simulink model "gm_uz_pmsm_model_3ph_dq"  (R2021b)
settings: Solver=FixedStepAuto  StartTime=0.0  StopTime=0.5  RelTol=1e-3
PreLoadFcn:
  | uz_pmsm_model_init_parameter
undefined symbols (not defined in the file or in its folder): friction_coefficient, inertia, k_i_d, k_p_d, k_p_q, L_d, L_q, polepair, psi_pm, R_1, setpoint_step, simulate_mechanical, simulate_open_loop, static_friction_torque, ts_regler
libraries: hdlmdlgenlib x69, dspsigops x18, slpidlib x2
(part 1 of 2)
settings Model: Creator=ts  LastModifiedBy=valen
settings SolverCC: AlgebraicLoopSolver=TrustRegion  AutoInsertRateTranBlk=on
settings DataIOCC: LimitDataPoints=on  SaveOutput=off  SaveTime=off
settings OptimizationCC: BlockReduction=off  ConditionallyExecuteInputs=off  DefaultParameterBehavior=Inlined  LifeSpan=inf
settings DebuggingCC: AlgebraicLoopMsg=error  InheritedTsInSrcMsg=none  SingleTaskRateTransMsg=error  AllowSymbolicDim=off  StrictBusMsg=ErrorOnBusTreatedAsVector  SFUnexpectedBacktrackingDiag=warning  SFNoUnconditionalDefaultTransitionDiag=warning  SFExecutionAtInitializationDiag=none  SFMachineParentedDataDiag=warning  ArithmeticOperatorsInVariantConditions=warning
settings HardwareCC: ProdBitPerPointer=32  ProdBitPerSizeT=32  ProdBitPerPtrDiffT=32  ProdLargestAtomicFloat=None  ProdIntDivRoundTo=Undefined  ProdEndianess=Unspecified  ProdWordSize=32  ProdHWDeviceType=ASIC/FPGA->ASIC/FPGA  ProdEqTarget=off
settings SFSimCC: SimUseLocalCustomCode=off  CustomCodeUndefinedFunction=UseInterfaceOnly
settings RTWCC: RTWUseLocalCustomCode=off
settings CodeAppCC: StateflowObjectComments=on
settings GRTTargetCC: TargetLangStandard=C89/C90 (ANSI)
settings ConfigComp: CovScope=ReferencedModels  CovMetricSettings=dw  CovSaveCumulativeToWorkspaceVar=on  CovSaveSingleToWorkspaceVar=on  CovExternalEMLEnable=off  CovSFcnEnable=off

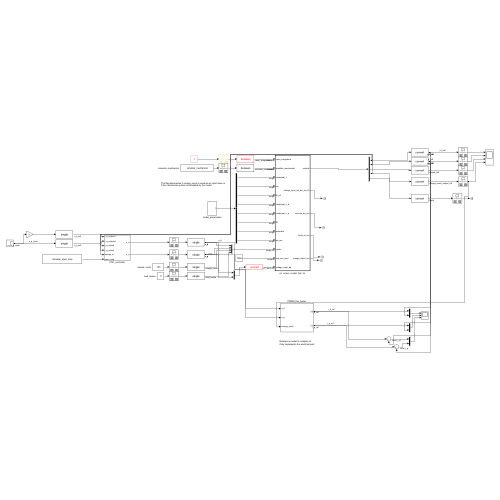
[thumbnail: Simulink's stored preview of the top-level diagram]
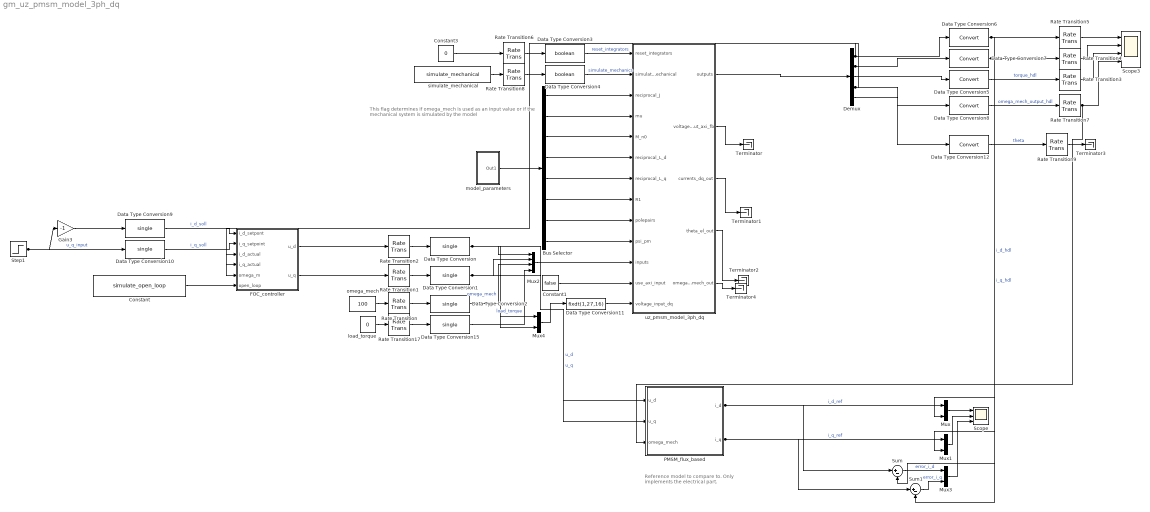
== system gm_uz_pmsm_model_3ph_dq ==
  note: This flag determines if omega_mech is used as an input value or
      | if the mechanical system is simulated by the model
  note: Reference model to compare to.
      | Only implements the electrical part.
  Bus Selector : BusSelector  OutputSignals=1_J,mu,M_R0,1_L_d,1_L_q,R_1,polepair,psi_pm
  Constant : Constant  Value=simulate_open_loop
  Constant1 : Constant  Value=false  OutDataTypeStr=boolean  SampleTime=-1
  Constant3 : Constant  Value=0
  Data Type Conversion{,1..2,9..10,15} (6 alike) : DataTypeConversion  OutDataTypeStr=single
  Data Type Conversion11 : DataTypeConversion  OutDataTypeStr=fixdt(1,27,16)
  Data Type Conversion{5..8,12} (5 alike) : DataTypeConversion
  Data Type Conversion3 : DataTypeConversion  OutDataTypeStr=boolean
  Data Type Conversion4 : DataTypeConversion  OutDataTypeStr=boolean
  Demux : Demux  Outputs=5
  FOC_controller : Subsystem
  Gain3 : Gain  Gain=-1
  Mux{,1,3..4} (4 alike) : Mux  Inputs=2
  Mux2 : Mux
  PMSM_flux_based : Subsystem
  Rate Transition{,1..2,6,8,17} (6 alike) : RateTransition  OutPortSampleTime=ts
  Rate Transition{3..5,7,9} (5 alike) : RateTransition
  Scope : Scope  NumInputPorts=3
  Scope3 : Scope  NumInputPorts=4
  Step1 : Step  Time=0.2  After=setpoint_step  SampleTime=ts_regler
  Sum : Sum  Inputs=|+-
  Sum1 : Sum  Inputs=|+-
  Terminator{,1..4} (5 alike) : Terminator
  load_torque : Constant  Value=0
  model_parameters : Subsystem
  omega_mech : Constant  Value=100
  simulate_mechanical : Constant  Value=simulate_mechanical
  uz_pmsm_model_3ph_dq : Subsystem  TreatAsAtomicUnit=on
  wires:
  uz_pmsm_model_3ph_dq/5(omega_mech_out) -> Terminator4/1
  Rate Transition9/1 -> Terminator3/1
  Data Type Conversion12/1 -> Rate Transition9/1  "theta"
  Demux/5 -> Data Type Conversion12/1
  uz_pmsm_model_3ph_dq/4(theta_el_out) -> Terminator2/1
  uz_pmsm_model_3ph_dq/3(currents_dq_out) -> Terminator1/1
  uz_pmsm_model_3ph_dq/2(voltage_input_dq_out_axi_fb) -> Terminator/1
  Data Type Conversion11/1 -> uz_pmsm_model_3ph_dq/13(voltage_input_dq)
  Mux4/1 -> Data Type Conversion11/1
  Constant1/1 -> uz_pmsm_model_3ph_dq/12(use_axi_input)
  Constant/1 -> FOC_controller/6(open_loop)
  omega_mech/1 -> Rate Transition/1
  FOC_controller/2(u_q) -> Rate Transition1/1
  FOC_controller/1(u_d) -> Rate Transition2/1
  Data Type Conversion10/1 -> FOC_controller/2(i_q_setpoint)  "i_q_soll"
  Data Type Conversion9/1 -> FOC_controller/1(i_d_setpont)  "i_d_soll"
  uz_pmsm_model_3ph_dq/1(outputs) -> Demux/1
  Mux2/1 -> uz_pmsm_model_3ph_dq/11(inputs)
  Data Type Conversion2/1 -> Mux2/3  "omega_mech"
  Data Type Conversion15/1 -> Mux2/4  "load_torque"
  Data Type Conversion1/1 -> Mux2/2, Mux4/2, PMSM_flux_based/2(u_q)  "u_q"
  Data Type Conversion/1 -> PMSM_flux_based/1(u_d), Mux4/1, Mux2/1  "u_d"
  Demux/2 -> Data Type Conversion7/1, FOC_controller/4(i_q_actual)
  Demux/4 -> FOC_controller/5(omega_m), Data Type Conversion8/1
  Demux/1 -> Data Type Conversion6/1, FOC_controller/3(i_d_actual)
  Gain3/1 -> Data Type Conversion9/1
  Demux/3 -> Data Type Conversion5/1
  Step1/1 -> Data Type Conversion10/1, Gain3/1  "u_q_input"
  Mux3/1 -> Scope/3
  Sum1/1 -> Mux3/2  "error_i_q"
  Sum/1 -> Mux3/1  "error_i_d"
  model_parameters/1(Out1) -> Bus Selector/1
  Bus Selector/8 -> uz_pmsm_model_3ph_dq/10(psi_pm)
  Bus Selector/7 -> uz_pmsm_model_3ph_dq/9(polepairs)
  Bus Selector/6 -> uz_pmsm_model_3ph_dq/8(R1)
  Bus Selector/5 -> uz_pmsm_model_3ph_dq/7(reciprocal_L_q)
  Bus Selector/4 -> uz_pmsm_model_3ph_dq/6(reciprocal_L_d)
  Bus Selector/3 -> uz_pmsm_model_3ph_dq/5(M_n0)
  Bus Selector/2 -> uz_pmsm_model_3ph_dq/4(mu)
  Bus Selector/1 -> uz_pmsm_model_3ph_dq/3(reciprocal_J)
  Rate Transition7/1 -> Scope3/4, PMSM_flux_based/3(omega_mech)
  Data Type Conversion8/1 -> Rate Transition7/1  "omega_mech_output_hdl"
  PMSM_flux_based/1(i_d) -> Sum/1, Mux/1  "i_d_ref"
  PMSM_flux_based/2(i_q) -> Sum1/1, Mux1/1  "i_q_ref"
  Mux1/1 -> Scope/2
  Mux/1 -> Scope/1
  Rate Transition17/1 -> Data Type Conversion15/1
  load_torque/1 -> Rate Transition17/1
  Data Type Conversion4/1 -> uz_pmsm_model_3ph_dq/2(simulate_mechanical)  "simulate_mechanics"
  Data Type Conversion3/1 -> uz_pmsm_model_3ph_dq/1(reset_integrators)  "reset_integrators"
  simulate_mechanical/1 -> Rate Transition8/1
  Rate Transition8/1 -> Data Type Conversion4/1
  Constant3/1 -> Rate Transition6/1
  Rate Transition6/1 -> Data Type Conversion3/1
  Rate Transition3/1 -> Scope3/3
  Rate Transition5/1 -> Scope3/1
  Rate Transition4/1 -> Scope3/2
  Data Type Conversion5/1 -> Rate Transition3/1  "torque_hdl"
  Data Type Conversion7/1 -> Mux1/2, Sum1/2, Rate Transition4/1  "i_q_hdl"
  Data Type Conversion6/1 -> Rate Transition5/1, Sum/2, Mux/2  "i_d_hdl"
  Rate Transition2/1 -> Data Type Conversion/1
  Rate Transition1/1 -> Data Type Conversion1/1
  Rate Transition/1 -> Data Type Conversion2/1

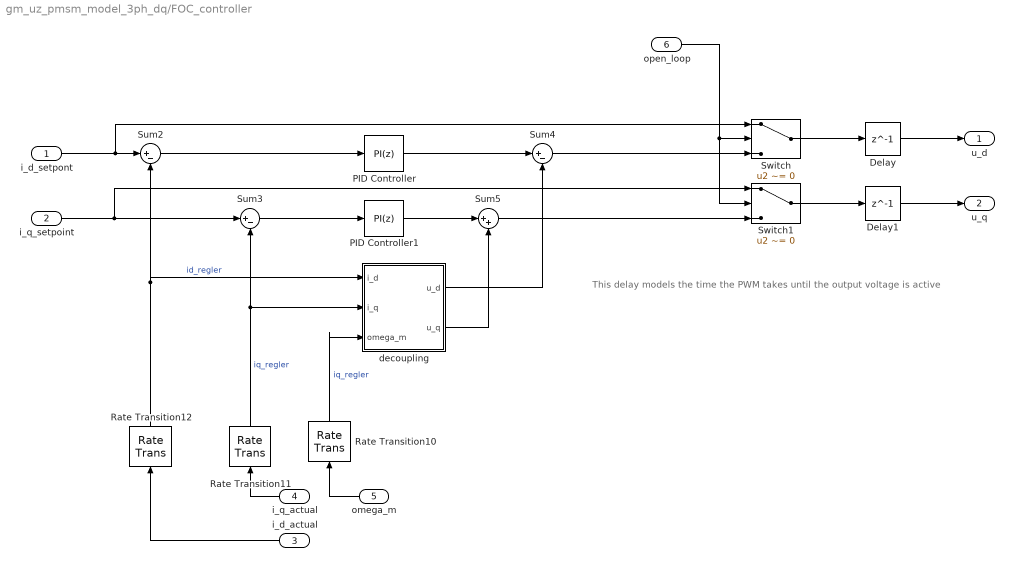
== system gm_uz_pmsm_model_3ph_dq/FOC_controller ==
  note: This delay models the time the PWM takes until the output voltage is active
  i_d_setpont : Inport
  i_q_setpoint : Inport  Port=2
  i_d_actual : Inport  Port=3
  i_q_actual : Inport  Port=4
  omega_m : Inport  Port=5
  open_loop : Inport  Port=6
  Delay : Delay  DelayLength=1
  Delay1 : Delay  DelayLength=1
  PID Controller : slpidlib/PID Controller  Controller=PI  Form=Parallel  TimeDomain=Discrete-time  UseExternalTs=off  SampleTime=-1  IntegratorMethod=Forward Euler  FilterMethod=Forward Euler  ControllerParametersSource=internal  P=k_p_d  I=k_i_d  D=0  UseFilter=on  N=100  TunerSelectOption=Transfer Function Based (PID Tuner App)  InitialConditionSource=internal  InitialConditionForIntegrator=0  InitialConditionForFilter=0  DifferentiatorICPrevScaledInput=0  ExternalReset=none  TrackingMode=off  Kt=1  LimitOutput=off  SatLimitsSource=internal  UpperSaturationLimit=inf  LowerSaturationLimit=-inf  LinearizeAsGain=on  AntiWindupMode=none  Kb=1  POutMin=[]  POutMax=[]  IOutMin=[]  IOutMax=[]  DOutMin=[]  DOutMax=[]  NOutMin=[]  NOutMax=[]  SumOutMin=[]  SumOutMax=[]  SaturationOutMin=[]  SaturationOutMax=[]  PParamMin=[]  PParamMax=[]  IParamMin=[]  IParamMax=[]  DParamMin=[]  DParamMax=[]  NParamMin=[]  NParamMax=[]  KbParamMin=[]  KbParamMax=[]  KtParamMin=[]  KtParamMax=[]  KbOutMin=[]  KbOutMax=[]  KtOutMin=[]  KtOutMax=[]  IntegratorOutMin=[]  IntegratorOutMax=[]  FilterOutMin=[]  FilterOutMax=[]  SumI1OutMin=[]  SumI1OutMax=[]  SumI2OutMin=[]  SumI2OutMax=[]  SumI3OutMin=[]  SumI3OutMax=[]  SumI4OutMin=[]  SumI4OutMax=[]  SumDOutMin=[]  SumDOutMax=[]  DifferentiatorOutMin=[]  DifferentiatorOutMax=[]  FilterDiffOutCoefMin=[]  FilterDiffOutCoefMax=[]  ReciprocalOutMin=[]  ReciprocalOutMax=[]  SumDenOutMin=[]  SumDenOutMax=[]  SumNumOutMin=[]  SumNumOutMax=[]  DivideOutMin=[]  DivideOutMax=[]  UdiffTsProdOutMin=[]  UdiffTsProdOutMax=[]  NTsProdOutMin=[]  NTsProdOutMax=[]  UintegralTsProdOutMin=[]  UintegralTsProdOutMax=[]  UngainTsProdOutMin=[]  UngainTsProdOutMax=[]  IntegratorContinuousStateAttributes=''  IntegratorStateMustResolveToSignalObject=off  IntegratorRTWStateStorageClass=Auto  FilterContinuousStateAttributes=''  FilterStateMustResolveToSignalObject=off  FilterRTWStateStorageClass=Auto  ParallelPVariant=InternalParameters  IdealPVariant=Disabled  IVariant=InternalParameters  DVariant=Disabled  IntegratorVariant=Discrete  SatVariant=Disabled  AWVariant=Passthrough  PCopyVariant=Disabled  TRVariant=Disabled  FdbkBlocksVariant=Forward  IdealPFdbkVariant=Disabled  SatFdbkVariant=Disabled  DerivativeFilterVariant=Disabled  NVariant=Disabled  NCopyVariant=Disabled_SignalSpec  FilterICVariant=Disabled  IntegratorICVariant=InternalICs  ExternalResetVariant=Disabled  TRSumVariant=Passthrough  SumFdbkVariant=Disabled  SumVariant=Sum_PI  TsampFilterVariant=InternalTs  TsampNgainVariant=Passthrough  TsampIntegralVariant=Passthrough  ExternalSaturationOutDataTypeStr=Inherit: Same as second input
  PID Controller1 : slpidlib/PID Controller  Controller=PI  Form=Parallel  TimeDomain=Discrete-time  UseExternalTs=off  SampleTime=-1  IntegratorMethod=Forward Euler  FilterMethod=Forward Euler  ControllerParametersSource=internal  P=k_p_q  I=k_i_d  D=0  UseFilter=on  N=100  TunerSelectOption=Transfer Function Based (PID Tuner App)  InitialConditionSource=internal  InitialConditionForIntegrator=0  InitialConditionForFilter=0  DifferentiatorICPrevScaledInput=0  ExternalReset=none  TrackingMode=off  Kt=1  LimitOutput=off  SatLimitsSource=internal  UpperSaturationLimit=inf  LowerSaturationLimit=-inf  LinearizeAsGain=on  AntiWindupMode=none  Kb=1  POutMin=[]  POutMax=[]  IOutMin=[]  IOutMax=[]  DOutMin=[]  DOutMax=[]  NOutMin=[]  NOutMax=[]  SumOutMin=[]  SumOutMax=[]  SaturationOutMin=[]  SaturationOutMax=[]  PParamMin=[]  PParamMax=[]  IParamMin=[]  IParamMax=[]  DParamMin=[]  DParamMax=[]  NParamMin=[]  NParamMax=[]  KbParamMin=[]  KbParamMax=[]  KtParamMin=[]  KtParamMax=[]  KbOutMin=[]  KbOutMax=[]  KtOutMin=[]  KtOutMax=[]  IntegratorOutMin=[]  IntegratorOutMax=[]  FilterOutMin=[]  FilterOutMax=[]  SumI1OutMin=[]  SumI1OutMax=[]  SumI2OutMin=[]  SumI2OutMax=[]  SumI3OutMin=[]  SumI3OutMax=[]  SumI4OutMin=[]  SumI4OutMax=[]  SumDOutMin=[]  SumDOutMax=[]  DifferentiatorOutMin=[]  DifferentiatorOutMax=[]  FilterDiffOutCoefMin=[]  FilterDiffOutCoefMax=[]  ReciprocalOutMin=[]  ReciprocalOutMax=[]  SumDenOutMin=[]  SumDenOutMax=[]  SumNumOutMin=[]  SumNumOutMax=[]  DivideOutMin=[]  DivideOutMax=[]  UdiffTsProdOutMin=[]  UdiffTsProdOutMax=[]  NTsProdOutMin=[]  NTsProdOutMax=[]  UintegralTsProdOutMin=[]  UintegralTsProdOutMax=[]  UngainTsProdOutMin=[]  UngainTsProdOutMax=[]  IntegratorContinuousStateAttributes=''  IntegratorStateMustResolveToSignalObject=off  IntegratorRTWStateStorageClass=Auto  FilterContinuousStateAttributes=''  FilterStateMustResolveToSignalObject=off  FilterRTWStateStorageClass=Auto  ParallelPVariant=InternalParameters  IdealPVariant=Disabled  IVariant=InternalParameters  DVariant=Disabled  IntegratorVariant=Discrete  SatVariant=Disabled  AWVariant=Passthrough  PCopyVariant=Disabled  TRVariant=Disabled  FdbkBlocksVariant=Forward  IdealPFdbkVariant=Disabled  SatFdbkVariant=Disabled  DerivativeFilterVariant=Disabled  NVariant=Disabled  NCopyVariant=Disabled_SignalSpec  FilterICVariant=Disabled  IntegratorICVariant=InternalICs  ExternalResetVariant=Disabled  TRSumVariant=Passthrough  SumFdbkVariant=Disabled  SumVariant=Sum_PI  TsampFilterVariant=InternalTs  TsampNgainVariant=Passthrough  TsampIntegralVariant=Passthrough  ExternalSaturationOutDataTypeStr=Inherit: Same as second input
  Rate Transition10 : RateTransition  OutPortSampleTime=ts_regler
  Rate Transition11 : RateTransition  OutPortSampleTime=ts_regler
  Rate Transition12 : RateTransition  OutPortSampleTime=ts_regler
  Sum2 : Sum  Inputs=|+-
  Sum3 : Sum  Inputs=|+-
  Sum4 : Sum  Inputs=|+-
  Sum5 : Sum  Inputs=|++
  Switch : Switch  Criteria=u2 ~= 0
  Switch1 : Switch  Criteria=u2 ~= 0
  decoupling : Subsystem
  u_d : Outport
  u_q : Outport  Port=2
  wires:
  Delay1/1 -> u_q/1
  Delay/1 -> u_d/1
  Switch1/1 -> Delay1/1
  Switch/1 -> Delay/1
  decoupling/2(u_q) -> Sum5/2
  decoupling/1(u_d) -> Sum4/2
  Rate Transition10/1 -> decoupling/3(omega_m)  "iq_regler"
  open_loop/1 -> Switch/2, Switch1/2
  i_q_setpoint/1 -> Sum3/1, Switch1/1
  Rate Transition11/1 -> Sum3/2, decoupling/2(i_q)  "iq_regler"
  Rate Transition12/1 -> Sum2/2, decoupling/1(i_d)  "id_regler"
  i_q_actual/1 -> Rate Transition11/1
  Sum3/1 -> PID Controller1/1
  omega_m/1 -> Rate Transition10/1
  Sum5/1 -> Switch1/3
  Sum2/1 -> PID Controller/1
  i_d_setpont/1 -> Sum2/1, Switch/1
  i_d_actual/1 -> Rate Transition12/1
  Sum4/1 -> Switch/3
  PID Controller1/1 -> Sum5/1
  PID Controller/1 -> Sum4/1

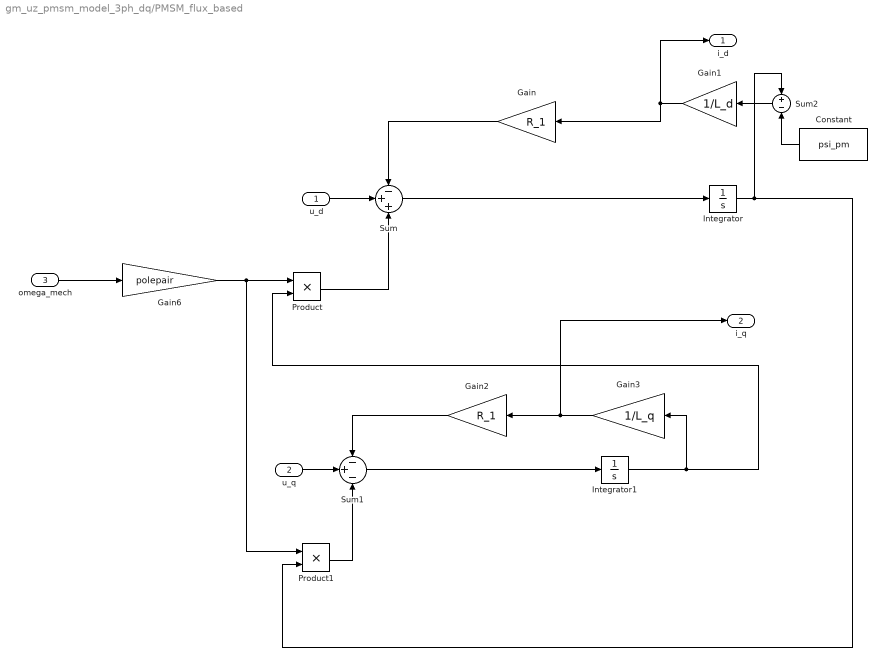
== system gm_uz_pmsm_model_3ph_dq/PMSM_flux_based ==
  u_d : Inport
  u_q : Inport  Port=2
  omega_mech : Inport  Port=3
  Constant : Constant  Value=psi_pm
  Gain : Gain  Gain=R_1
  Gain1 : Gain  Gain=1/L_d
  Gain2 : Gain  Gain=R_1
  Gain3 : Gain  Gain=1/L_q
  Gain6 : Gain  Gain=polepair
  Integrator : Integrator
  Integrator1 : Integrator
  Product : Product
  Product1 : Product
  Sum : Sum  Inputs=-++
  Sum1 : Sum  Inputs=-+-
  Sum2 : Sum  Inputs=+-
  i_d : Outport
  i_q : Outport  Port=2
  wires:
  omega_mech/1 -> Gain6/1
  Gain3/1 -> Gain2/1, i_q/1
  Gain2/1 -> Sum1/1
  Sum1/1 -> Integrator1/1
  Product1/1 -> Sum1/3
  Integrator1/1 -> Product/2, Gain3/1
  Product/1 -> Sum/3
  Gain6/1 -> Product/1, Product1/1
  Gain1/1 -> i_d/1, Gain/1
  Sum2/1 -> Gain1/1
  Constant/1 -> Sum2/2
  Integrator/1 -> Sum2/1, Product1/2
  Gain/1 -> Sum/1
  Sum/1 -> Integrator/1
  u_q/1 -> Sum1/2
  u_d/1 -> Sum/2

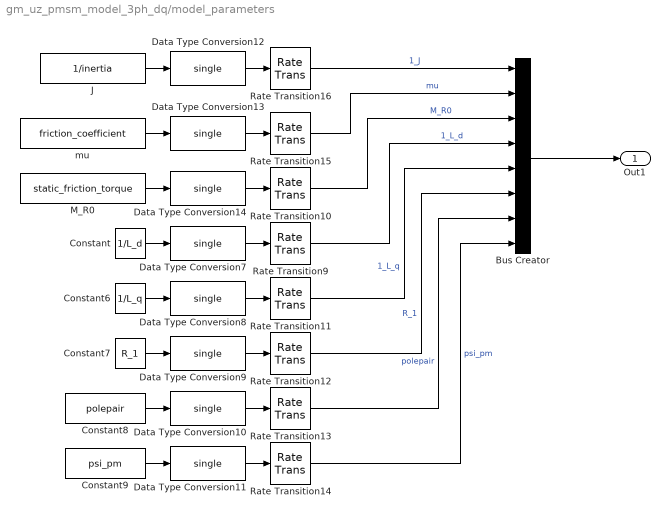
== system gm_uz_pmsm_model_3ph_dq/model_parameters ==
  Bus Creator : BusCreator  Inputs=8
  Constant : Constant  Value=1/L_d
  Constant6 : Constant  Value=1/L_q
  Constant7 : Constant  Value=R_1
  Constant8 : Constant  Value=polepair
  Constant9 : Constant  Value=psi_pm
  Data Type Conversion{7..14} (8 alike) : DataTypeConversion  OutDataTypeStr=single
  J : Constant  Value=1/inertia
  M_R0 : Constant  Value=static_friction_torque
  Rate Transition{9..16} (8 alike) : RateTransition  OutPortSampleTime=ts
  mu : Constant  Value=friction_coefficient
  Out1 : Outport
  wires:
  Constant/1 -> Data Type Conversion7/1
  Constant9/1 -> Data Type Conversion11/1
  Constant7/1 -> Data Type Conversion9/1
  Data Type Conversion13/1 -> Rate Transition15/1
  Rate Transition11/1 -> Bus Creator/5  "1_L_q"
  M_R0/1 -> Data Type Conversion14/1
  mu/1 -> Data Type Conversion13/1
  Data Type Conversion10/1 -> Rate Transition13/1
  Data Type Conversion8/1 -> Rate Transition11/1
  J/1 -> Data Type Conversion12/1
  Rate Transition9/1 -> Bus Creator/4  "1_L_d"
  Constant6/1 -> Data Type Conversion8/1
  Rate Transition15/1 -> Bus Creator/2  "mu"
  Data Type Conversion9/1 -> Rate Transition12/1
  Constant8/1 -> Data Type Conversion10/1
  Data Type Conversion11/1 -> Rate Transition14/1
  Bus Creator/1 -> Out1/1
  Rate Transition13/1 -> Bus Creator/7  "polepair"
  Rate Transition16/1 -> Bus Creator/1  "1_J"
  Rate Transition12/1 -> Bus Creator/6  "R_1"
  Data Type Conversion14/1 -> Rate Transition10/1
  Rate Transition14/1 -> Bus Creator/8  "psi_pm"
  Rate Transition10/1 -> Bus Creator/3  "M_R0"
  Data Type Conversion7/1 -> Rate Transition9/1
  Data Type Conversion12/1 -> Rate Transition16/1

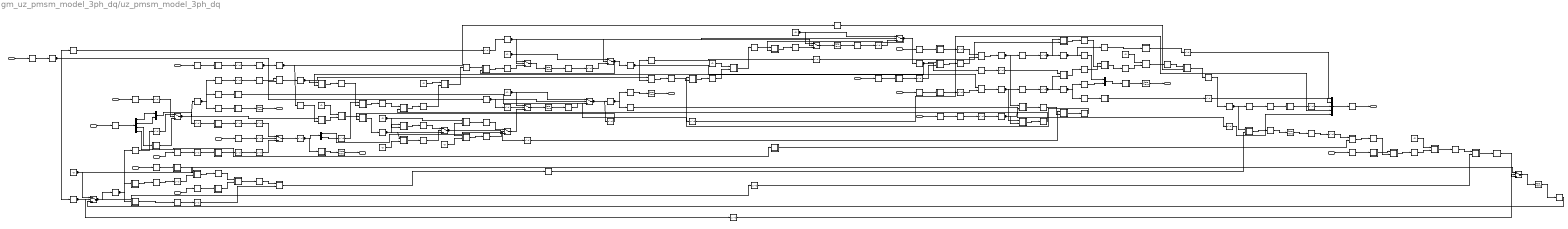
== system gm_uz_pmsm_model_3ph_dq/uz_pmsm_model_3ph_dq ==
  note: https://de.mathworks.com/help/releases/R2021a/hdlcoder/ug/troubleshoot-generate-implementation-model-from-simscape-pmsm.html?searchHighlight=troubleshoot-generate-implementation-model-from-simscape-pmsm&s_tid=doc_srchtitle
  reset_integrators : Inport  OutDataTypeStr=boolean  PortDimensions=1  SampleTime=1e-06
  simulate_mechanical : Inport  Port=2  OutDataTypeStr=boolean  PortDimensions=1  SampleTime=1e-06
  reciprocal_J : Inport  Port=3  OutDataTypeStr=single  PortDimensions=1  SampleTime=1e-06
  mu : Inport  Port=4  OutDataTypeStr=single  PortDimensions=1  SampleTime=1e-06
  M_n0 : Inport  Port=5  OutDataTypeStr=single  PortDimensions=1  SampleTime=1e-06
  reciprocal_L_d : Inport  Port=6  OutDataTypeStr=single  PortDimensions=1  SampleTime=1e-06
  reciprocal_L_q : Inport  Port=7  OutDataTypeStr=single  PortDimensions=1  SampleTime=1e-06
  R1 : Inport  Port=8  OutDataTypeStr=single  PortDimensions=1  SampleTime=1e-06
  polepairs : Inport  Port=9  OutDataTypeStr=single  PortDimensions=1  SampleTime=1e-06
  psi_pm : Inport  Port=10  OutDataTypeStr=single  PortDimensions=1  SampleTime=1e-06
  inputs : Inport  Port=11  OutDataTypeStr=single  PortDimensions=[4]  SampleTime=1e-06
  use_axi_input : Inport  Port=12  OutDataTypeStr=boolean  PortDimensions=1  SampleTime=1e-06
  voltage_input_dq : Inport  Port=13  OutDataTypeStr=fixdt(1, 27, 16)  PortDimensions=[2]  SampleTime=1e-06
  Abs : Subsystem
      mask Display: disp('NFP\nabs');
  Abs_outbuff : hdlmdlgenlib/Buffer
      settings: SourceProductBaseCode=SL
  Compare To Constant1_const : Constant  Value=double(-3.1415927410125732)  OutDataTypeStr=double  SampleTime=1e-08
  Compare To Constant1_relop : Subsystem
      mask Display: disp('NFP\nrelop');
  Compare To Constant1_relop_outbuff : hdlmdlgenlib/Buffer
      settings: SourceProductBaseCode=SL
  Compare To Constant_const : Constant  Value=double(3.1415927410125732)  OutDataTypeStr=double  SampleTime=1e-08
  Compare To Constant_relop : Subsystem
      mask Display: disp('NFP\nrelop');
  Compare To Constant_relop_outbuff : hdlmdlgenlib/Buffer
      settings: SourceProductBaseCode=SL
  Constant : Constant  Value=double(6.283185307179586)  OutDataTypeStr=double  SampleTime=1e-08
  Data Type Conversion1 : Subsystem
      mask Display: disp('NFP\nconv');
  Data Type Conversion10 : Subsystem
      mask Display: disp('NFP\nconv');
  Data Type Conversion10_out1 : hdlmdlgenlib/Buffer
      settings: SourceProductBaseCode=SL
  Data Type Conversion10_out1_in_pipe : Delay  DelayLength=double(7)  InitialCondition=0  SampleTime=1e-08
  Data Type Conversion11 : Subsystem
      mask Display: disp('NFP\nconv');
  Data Type Conversion12 : Subsystem
      mask Display: disp('NFP\nconv');
  Data Type Conversion13 : Subsystem
      mask Display: disp('NFP\nconv');
  Data Type Conversion14 : Subsystem
      mask Display: disp('NFP\nconv');
  Data Type Conversion15 : Subsystem
      mask Display: disp('NFP\nconv');
  Data Type Conversion16 : Subsystem
      mask Display: disp('NFP\nconv');
  Data Type Conversion17 : Subsystem
      mask Display: disp('NFP\nconv');
  Data Type Conversion18 : Subsystem
      mask Display: disp('NFP\nconv');
  Data Type Conversion18_in_pipe : Delay  DelayLength=double(10)  InitialCondition=0  SampleTime=1e-08
  Data Type Conversion18_out_pipe : Delay  DelayLength=double(7)  InitialCondition=0  SampleTime=1e-08
  Data Type Conversion19 : Subsystem
      mask Display: disp('NFP\nconv');
  Data Type Conversion1_in_pipe : Delay  DelayLength=double(10)  InitialCondition=0  SampleTime=1e-08
  Data Type Conversion1_out_pipe : Delay  DelayLength=double(7)  InitialCondition=0  SampleTime=1e-08
  Data Type Conversion2 : Subsystem
      mask Display: disp('NFP\nconv');
  Data Type Conversion20 : Subsystem
      mask Display: disp('NFP\nconv');
  Data Type Conversion21 : Subsystem
      mask Display: disp('NFP\nconv');
  Data Type Conversion3 : Subsystem
      mask Display: disp('NFP\nconv');
  Data Type Conversion4 : Subsystem
      mask Display: disp('NFP\nconv');
  Data Type Conversion5 : Subsystem
      mask Display: disp('NFP\nconv');
  Data Type Conversion6 : Subsystem
      mask Display: disp('NFP\nconv');
  Data Type Conversion6_out1 : hdlmdlgenlib/Buffer
      settings: SourceProductBaseCode=SL
  Data Type Conversion6_out1_in_pipe : Delay  DelayLength=double(7)  InitialCondition=0  SampleTime=1e-08
  Data Type Conversion7 : Subsystem
      mask Display: disp('NFP\nconv');
  Data Type Conversion7_out1_in_pipe : Delay  DelayLength=double(7)  InitialCondition=0  SampleTime=1e-08
  Data Type Conversion8 : Subsystem
      mask Display: disp('NFP\nconv');
  Data Type Conversion8_out1_in_pipe : Delay  DelayLength=double(7)  InitialCondition=0  SampleTime=1e-08
  Data Type Conversion9 : Subsystem
      mask Display: disp('NFP\nconv');
  Data Type Conversion9_out1_in_pipe : Delay  DelayLength=double(7)  InitialCondition=0  SampleTime=1e-08
  Delay : RateTransition  OutPortSampleTimeOpt=Multiple of input port sample time  OutPortSampleTimeMultiple=100
  Delay1_lowered{,1..3} (4 alike) : RateTransition  OutPortSampleTimeOpt=Multiple of input port sample time  OutPortSampleTimeMultiple=100
  Factor : Subsystem
      mask Display: disp('NFP\nmul');
  Factor_const : Constant  Value=double(1.5)  OutDataTypeStr=double  SampleTime=1e-08
  Factor_outbuff : hdlmdlgenlib/Buffer
      settings: SourceProductBaseCode=SL
  From{,1..12} (13 alike) : hdlmdlgenlib/Buffer
      settings: SourceProductBaseCode=SL
  Gain : Subsystem
      mask Display: disp('NFP\nmul');
  Gain1 : Subsystem
      mask Display: disp('NFP\nmul');
  Gain2 : Subsystem
      mask Display: disp('NFP\nmul');
  Gain3 : Subsystem
      mask Display: disp('NFP\nmul');
  Gain_const{,1..3} (4 alike) : Constant  Value=double(1e-06)  OutDataTypeStr=double  SampleTime=1e-08
  Gain_outbuff : hdlmdlgenlib/Buffer
      settings: SourceProductBaseCode=SL
  Gain_outbuff1 : hdlmdlgenlib/Buffer
      settings: SourceProductBaseCode=SL
  Gain_outbuff2 : hdlmdlgenlib/Buffer
      settings: SourceProductBaseCode=SL
  Goto{,1..5} (6 alike) : hdlmdlgenlib/Buffer
      settings: SourceProductBaseCode=SL
  Initial_Val{,1..3} (4 alike) : Constant  Value=double(0)  OutDataTypeStr=double  SampleTime=1e-08
  M_Mi : hdlmdlgenlib/Buffer
      settings: SourceProductBaseCode=SL
  Mux_in_pipe{0..4} (5 alike) : Delay  DelayLength=double(7)  InitialCondition=0  SampleTime=1e-08
  Product : Subsystem
      mask Display: disp('NFP\nmul');
  Product1 : Subsystem
      mask Display: disp('NFP\nmul');
  Product10 : Subsystem
      mask Display: disp('NFP\nmul');
  Product10_outbuff : hdlmdlgenlib/Buffer
      settings: SourceProductBaseCode=SL
  Product11 : Subsystem
      mask Display: disp('NFP\nmul');
  Product11_outbuff : hdlmdlgenlib/Buffer
      settings: SourceProductBaseCode=SL
  Product12 : Subsystem
      mask Display: disp('NFP\nmul');
  Product12_outbuff : hdlmdlgenlib/Buffer
      settings: SourceProductBaseCode=SL
  Product1_outbuff : hdlmdlgenlib/Buffer
      settings: SourceProductBaseCode=SL
  Product2 : Subsystem
      mask Display: disp('NFP\nmul');
  Product2_outbuff : hdlmdlgenlib/Buffer
      settings: SourceProductBaseCode=SL
  Product3 : Subsystem
      mask Display: disp('NFP\nmul');
  Product31 : Subsystem
      mask Display: disp('NFP\nmul');
  Product3_outbuff : hdlmdlgenlib/Buffer
      settings: SourceProductBaseCode=SL
  Product4 : Subsystem
      mask Display: disp('NFP\nmul');
  Product4_outbuff : hdlmdlgenlib/Buffer
      settings: SourceProductBaseCode=SL
  Product5 : Subsystem
      mask Display: disp('NFP\nmul');
  Product5_outbuff : hdlmdlgenlib/Buffer
      settings: SourceProductBaseCode=SL
  Product6 : Subsystem
      mask Display: disp('NFP\nmul');
  Product6_outbuff : hdlmdlgenlib/Buffer
      settings: SourceProductBaseCode=SL
  Product7 : Subsystem
      mask Display: disp('NFP\nmul');
  Product7_outbuff : hdlmdlgenlib/Buffer
      settings: SourceProductBaseCode=SL
  Product8 : Subsystem
      mask Display: disp('NFP\nmul');
  Product8_outbuff : hdlmdlgenlib/Buffer
      settings: SourceProductBaseCode=SL
  Product9 : Subsystem
      mask Display: disp('NFP\nmul');
  Product9_outbuff : hdlmdlgenlib/Buffer
      settings: SourceProductBaseCode=SL
  Product_outbuff : hdlmdlgenlib/Buffer
      settings: SourceProductBaseCode=SL
  Sign1 : Subsystem
      mask Display: disp('NFP\nsignum');
  Sign1_outbuff : hdlmdlgenlib/Buffer
      settings: SourceProductBaseCode=SL
  Sum : Subsystem
      mask Display: disp('NFP\nadd');
  Sum1 : Subsystem
      mask Display: disp('NFP\nadd');
  Sum11 : Subsystem
      mask Display: disp('NFP\nadd');
  Sum1_outbuff : hdlmdlgenlib/Buffer
      settings: SourceProductBaseCode=SL
  Sum1_outbuff1 : hdlmdlgenlib/Buffer
      settings: SourceProductBaseCode=SL
  Sum1_stage2 : Subsystem
      mask Display: disp('NFP\nadd');
  Sum1_stage2_outbuff : hdlmdlgenlib/Buffer
      settings: SourceProductBaseCode=SL
  Sum1_stage3 : Subsystem
      mask Display: disp('NFP\nadd');
  Sum1_stage3_outbuff : hdlmdlgenlib/Buffer
      settings: SourceProductBaseCode=SL
  Sum2 : Subsystem
      mask Display: disp('NFP\nadd');
  Sum21 : Subsystem
      mask Display: disp('NFP\nadd');
  Sum2_outbuff : hdlmdlgenlib/Buffer
      settings: SourceProductBaseCode=SL
  Sum2_outbuff1 : hdlmdlgenlib/Buffer
      settings: SourceProductBaseCode=SL
  Sum3 : Subsystem
      mask Display: disp('NFP\nadd');
  Sum31 : Subsystem
      mask Display: disp('NFP\nadd');
  Sum32 : Subsystem
      mask Display: disp('NFP\nadd');
  Sum33 : Subsystem
      mask Display: disp('NFP\nadd');
  Sum3_outbuff{,1..3} (4 alike) : hdlmdlgenlib/Buffer
      settings: SourceProductBaseCode=SL
  Sum4 : Subsystem
      mask Display: disp('NFP\nadd');
  Sum5 : Subsystem
      mask Display: disp('NFP\nadd');
  Sum5_outbuff : hdlmdlgenlib/Buffer
      settings: SourceProductBaseCode=SL
  Sum_outbuff : hdlmdlgenlib/Buffer
      settings: SourceProductBaseCode=SL
  Sum_outbuff1 : hdlmdlgenlib/Buffer
      settings: SourceProductBaseCode=SL
  Sum_stage2 : Subsystem
      mask Display: disp('NFP\nadd');
  Sum_stage2_outbuff : hdlmdlgenlib/Buffer
      settings: SourceProductBaseCode=SL
  Sum_stage3 : Subsystem
      mask Display: disp('NFP\nadd');
  Sum_stage3_outbuff : hdlmdlgenlib/Buffer
      settings: SourceProductBaseCode=SL
  Switch{,1..2,11} (4 alike) : Switch  Criteria=u2 ~= 0  Threshold=double(0)  OutDataTypeStr=double  SampleTime=1e-08
  Switch2_in_pipe0 : Delay  DelayLength=double(10)  InitialCondition=0  SampleTime=1e-08
  Switch2_in_pipe1 : Delay  DelayLength=double(10)  InitialCondition=0  SampleTime=1e-08
  Switch2_in_pipe2 : Delay  DelayLength=double(10)  InitialCondition=0  SampleTime=1e-08
  Switch2_out_pipe : Delay  DelayLength=double(10)  InitialCondition=0  SampleTime=1e-08
  delayMatch{,1..10} (11 alike) : Delay  DelayLength=double(1)  InitialCondition=0  SampleTime=1e-08
  i_d : hdlmdlgenlib/Buffer
      settings: SourceProductBaseCode=SL
  i_d_out_pipe : Delay  DelayLength=double(10)  InitialCondition=0  SampleTime=1e-08
  i_q : hdlmdlgenlib/Buffer
      settings: SourceProductBaseCode=SL
  i_q_out_pipe : Delay  DelayLength=double(10)  InitialCondition=0  SampleTime=1e-08
  in0_repeat : dspsigops/Repeat  N=double(100)  RateOptions=Allow multirate processing  ic=0  mode=Unused parameter value
  in10_repeat : dspsigops/Repeat  N=double(100)  RateOptions=Allow multirate processing  ic=0  mode=Unused parameter value
  in11_repeat : dspsigops/Repeat  N=double(100)  RateOptions=Allow multirate processing  ic=0  mode=Unused parameter value
  in12_repeat : dspsigops/Repeat  N=double(100)  RateOptions=Allow multirate processing  ic=0  mode=Unused parameter value
  in13_repeat : dspsigops/Repeat  N=double(100)  RateOptions=Allow multirate processing  ic=0  mode=Unused parameter value
  in14_repeat : dspsigops/Repeat  N=double(100)  RateOptions=Allow multirate processing  ic=0  mode=Unused parameter value
  in15_repeat : dspsigops/Repeat  N=double(100)  RateOptions=Allow multirate processing  ic=0  mode=Unused parameter value
  in16_repeat : dspsigops/Repeat  N=double(100)  RateOptions=Allow multirate processing  ic=0  mode=Unused parameter value
  in17_repeat : dspsigops/Repeat  N=double(100)  RateOptions=Allow multirate processing  ic=0  mode=Unused parameter value
  in1_repeat : dspsigops/Repeat  N=double(100)  RateOptions=Allow multirate processing  ic=0  mode=Unused parameter value
  in2_repeat : dspsigops/Repeat  N=double(100)  RateOptions=Allow multirate processing  ic=0  mode=Unused parameter value
  in3_repeat : dspsigops/Repeat  N=double(100)  RateOptions=Allow multirate processing  ic=0  mode=Unused parameter value
  in4_repeat : dspsigops/Repeat  N=double(100)  RateOptions=Allow multirate processing  ic=0  mode=Unused parameter value
  in5_repeat : dspsigops/Repeat  N=double(100)  RateOptions=Allow multirate processing  ic=0  mode=Unused parameter value
  in6_repeat : dspsigops/Repeat  N=double(100)  RateOptions=Allow multirate processing  ic=0  mode=Unused parameter value
  in7_repeat : dspsigops/Repeat  N=double(100)  RateOptions=Allow multirate processing  ic=0  mode=Unused parameter value
  in8_repeat : dspsigops/Repeat  N=double(100)  RateOptions=Allow multirate processing  ic=0  mode=Unused parameter value
  in9_repeat : dspsigops/Repeat  N=double(100)  RateOptions=Allow multirate processing  ic=0  mode=Unused parameter value
  integrator1_out1 : hdlmdlgenlib/Buffer
      settings: SourceProductBaseCode=SL
  mechanical_system_out1 : hdlmdlgenlib/Buffer
      settings: SourceProductBaseCode=SL
  mux : Mux  Inputs=2
  mux1 : Mux  Inputs=2
  mux2 : Mux  Inputs=5
  omega : hdlmdlgenlib/Buffer
      settings: SourceProductBaseCode=SL
  omega_in_pipe : Delay  DelayLength=double(10)  InitialCondition=0  SampleTime=1e-08
  pmsm_out3 : hdlmdlgenlib/Buffer
      settings: SourceProductBaseCode=SL
  pmsm_out3_out_pipe : Delay  DelayLength=double(10)  InitialCondition=0  SampleTime=1e-08
  pmsm_out4 : hdlmdlgenlib/Buffer
      settings: SourceProductBaseCode=SL
  pmsm_out4_out_pipe : Delay  DelayLength=double(10)  InitialCondition=0  SampleTime=1e-08
  psi_d : hdlmdlgenlib/Buffer
      settings: SourceProductBaseCode=SL
  psi_q : hdlmdlgenlib/Buffer
      settings: SourceProductBaseCode=SL
  reset_in{,1..3} (4 alike) : Switch  Criteria=u2 ~= 0  Threshold=double(0)  OutDataTypeStr=double  SampleTime=1e-08
  reset_integrators1 : hdlmdlgenlib/Buffer
      settings: SourceProductBaseCode=SL
  reset_integrators_in_pipe : Delay  DelayLength=double(10)  InitialCondition=0  SampleTime=1e-08
  reset_out{,1..3} (4 alike) : Switch  Criteria=u2 ~= 0  Threshold=double(0)  OutDataTypeStr=double  SampleTime=1e-08
  t : Demux
  t1 : Demux  Outputs=2
  t{2..5} (4 alike) : RateTransition  OutPortSampleTimeOpt=Multiple of input port sample time  OutPortSampleTimeMultiple=100
  t6 : DownSample  N=double(100)  phase=double(90)  RateOptions=Allow multirate processing
  theta_el : hdlmdlgenlib/Buffer
      settings: SourceProductBaseCode=SL
  u_d_in_pipe : Delay  DelayLength=double(10)  InitialCondition=0  SampleTime=1e-08
  u_q_in_pipe : Delay  DelayLength=double(10)  InitialCondition=0  SampleTime=1e-08
  outputs : Outport  SampleTime=1e-06
  voltage_input_dq_out_axi_fb : Outport  Port=2  SampleTime=1e-06
  currents_dq_out : Outport  Port=3  SampleTime=1e-06
  theta_el_out : Outport  Port=4  SampleTime=1e-06
  omega_mech_out : Outport  Port=5  SampleTime=1e-06
  wires:
  reset_integrators/1 -> in9_repeat/1
  simulate_mechanical/1 -> in12_repeat/1
  reciprocal_J/1 -> in5_repeat/1
  mu/1 -> in3_repeat/1
  M_n0/1 -> in4_repeat/1
  reciprocal_L_d/1 -> in1_repeat/1
  reciprocal_L_q/1 -> in14_repeat/1
  R1/1 -> in0_repeat/1
  polepairs/1 -> in11_repeat/1
  psi_pm/1 -> in2_repeat/1
  inputs/1 -> in7_repeat/1
  use_axi_input/1 -> in16_repeat/1
  voltage_input_dq/1 -> in17_repeat/1
  t6/1 -> outputs/1
  t2/1 -> currents_dq_out/1
  t3/1 -> omega_mech_out/1
  t4/1 -> theta_el_out/1
  t5/1 -> voltage_input_dq_out_axi_fb/1
  Delay1_lowered/1 -> in15_repeat/1
  Delay1_lowered1/1 -> in13_repeat/1
  Delay1_lowered2/1 -> in10_repeat/1
  Delay/1 -> in6_repeat/1
  Delay1_lowered3/1 -> in8_repeat/1
  reset_in3/1 -> Delay1_lowered/1
  reset_in2/1 -> Delay1_lowered1/1
  reset_in1/1 -> Delay1_lowered2/1
  Sum_outbuff/1 -> Delay/1
  reset_in/1 -> Delay1_lowered3/1
  in0_repeat/1 -> Data Type Conversion6/1(In1)
  in1_repeat/1 -> Data Type Conversion7/1(In1)
  in2_repeat/1 -> Data Type Conversion9/1(In1)
  in3_repeat/1 -> Data Type Conversion12/1(In1)
  in4_repeat/1 -> Data Type Conversion13/1(In1)
  in5_repeat/1 -> Data Type Conversion14/1(In1)
  in6_repeat/1 -> delayMatch8/1
  in7_repeat/1 -> t/1
  in8_repeat/1 -> reset_out/3
  in9_repeat/1 -> Goto/1
  in10_repeat/1 -> reset_out1/3
  in11_repeat/1 -> Data Type Conversion10/1(In1)
  in12_repeat/1 -> delayMatch5/1
  in13_repeat/1 -> delayMatch1/1
  in14_repeat/1 -> Data Type Conversion8/1(In1)
  in15_repeat/1 -> delayMatch/1
  in16_repeat/1 -> Switch2_in_pipe1/1
  in17_repeat/1 -> Data Type Conversion18_in_pipe/1
  From3/1 -> Data Type Conversion15/1(In1)
  Sum2_outbuff/1 -> Product5/2(In2)
  Product5_outbuff/1 -> Product8/1(In1), i_d/1
  i_d_out_pipe/1 -> Product2/1(In1), Goto1/1
  Product2_outbuff/1 -> Sum32/2(In2)
  From12/1 -> Data Type Conversion21/1(In1)
  From11/1 -> Data Type Conversion17/1(In1)
  theta_el/1 -> Data Type Conversion20/1(In1), Data Type Conversion2/1(In1)
  delayMatch4/1 -> Switch11/1
  delayMatch6/1 -> Product12/2(In2)
  Product12_outbuff/1 -> Sum5/1(In1)
  Sum5_outbuff/1 -> Product4/1(In1)
  delayMatch7/1 -> Product4/2(In2)
  integrator1_out1/1 -> Sign1/1(In1), Abs/1(In1), mechanical_system_out1/1
  Initial_Val/1 -> reset_out/1, reset_in/1
  mux/1 -> Data Type Conversion1_in_pipe/1
  Sum1_outbuff/1 -> Product11/2(In2)
  Product11_outbuff/1 -> Gain/2(In2)
  Gain_outbuff/1 -> Sum3/1(In1)
  Sum3_outbuff/1 -> reset_in/3
  delayMatch9/1 -> Sum3/2(In2)
  delayMatch10/1 -> reset_in/2
  From/1 -> reset_integrators_in_pipe/1
  Goto/1 -> From2/1, From1/1, From/1
  Initial_Val1/1 -> reset_out1/1, reset_in1/1
  Switch1/1 -> reset_in1/3
  Sum1_outbuff1/1 -> Switch/1
  Constant/1 -> Sum21/1(In1), Sum11/2(In2)
  Sum2_outbuff1/1 -> Switch1/1
  Goto4/1 -> From9/1, From8/1
  Goto5/1 -> From12/1, From11/1, From10/1
  From10/1 -> omega_in_pipe/1
  omega/1 -> Product10/1(In1)
  Product10_outbuff/1 -> Product3/1(In1), Product1/1(In1)
  Initial_Val2/1 -> reset_out2/1, reset_in2/1
  Sum3_outbuff1/1 -> reset_in2/3
  Gain_outbuff1/1 -> Sum31/1(In1)
  Sum1_stage3_outbuff/1 -> Gain2/2(In2)
  Product6_outbuff/1 -> Product7/1(In1), i_q/1
  i_q_out_pipe/1 -> Product31/2(In2), Goto2/1
  Goto2/1 -> From5/1, From3/1
  mux1/1 -> Data Type Conversion3/1(In1)
  From6/1 -> mux1/1
  Goto1/1 -> From6/1, From4/1
  From4/1 -> Data Type Conversion11/1(In1)
  From7/1 -> Data Type Conversion16/1(In1)
  Goto3/1 -> From7/1
  M_Mi/1 -> Sum/1(In1), Goto3/1
  Product9_outbuff/1 -> M_Mi/1
  Factor_outbuff/1 -> Product9/1(In1)
  Sum3_outbuff2/1 -> Factor/2(In2)
  Initial_Val3/1 -> reset_out3/1, reset_in3/1
  Sum3_outbuff3/1 -> reset_in3/3
  Gain_outbuff2/1 -> Sum33/1(In1)
  Sum_stage3_outbuff/1 -> Gain3/2(In2)
  Data Type Conversion18_out_pipe/1 -> Switch2_in_pipe2/1
  Switch2_out_pipe/1 -> Data Type Conversion19/1(In1), t1/1
  Data Type Conversion1_out_pipe/1 -> Switch2_in_pipe0/1
  delayMatch1/1 -> reset_out2/3
  delayMatch/1 -> reset_out3/3
  i_d/1 -> i_d_out_pipe/1
  pmsm_out4/1 -> pmsm_out4_out_pipe/1
  i_q/1 -> i_q_out_pipe/1
  mux2/1 -> t6/1
  pmsm_out3/1 -> pmsm_out3_out_pipe/1
  Switch2/1 -> Switch2_out_pipe/1
  Data Type Conversion6_out1_in_pipe/1 -> Data Type Conversion6_out1/1
  Data Type Conversion7_out1_in_pipe/1 -> Product5/1(In1)
  Data Type Conversion9_out1_in_pipe/1 -> Sum2/2(In2)
  reset_integrators_in_pipe/1 -> reset_integrators1/1
  Data Type Conversion10_out1_in_pipe/1 -> Data Type Conversion10_out1/1
  omega_in_pipe/1 -> omega/1
  u_q_in_pipe/1 -> Sum1_stage2/1(In1)
  Data Type Conversion8_out1_in_pipe/1 -> Product6/2(In2)
  Mux_in_pipe2/1 -> mux2/3
  u_d_in_pipe/1 -> Sum_stage2/1(In1)
  Data Type Conversion18_in_pipe/1 -> Data Type Conversion18/1(In1)
  Switch2_in_pipe0/1 -> Switch2/1
  Switch2_in_pipe2/1 -> Switch2/3
  Data Type Conversion1_in_pipe/1 -> Data Type Conversion1/1(In1)
  t/1 -> mux/1
  t/2 -> mux/2
  t/3 -> Data Type Conversion4/1(In1)
  t/4 -> Data Type Conversion5/1(In1)
  Compare To Constant1_const/1 -> Compare To Constant1_relop/2(In2)
  Compare To Constant_const/1 -> Compare To Constant_relop/2(In2)
  Sum1_stage2_outbuff/1 -> Sum1_stage3/1(In1)
  Sum_stage2_outbuff/1 -> Sum_stage3/1(In1)
  t1/1 -> u_d_in_pipe/1
  t1/2 -> u_q_in_pipe/1
  Gain_const/1 -> Gain/1(In1)
  Gain_const1/1 -> Gain1/1(In1)
  Gain_const2/1 -> Gain2/1(In1)
  Factor_const/1 -> Factor/1(In1)
  Gain_const3/1 -> Gain3/1(In1)
  Switch2_in_pipe1/1 -> Switch2/2
  Product8_outbuff/1 -> Sum_stage2/2(In2)
  Product_outbuff/1 -> Sum_stage3/2(In2)
  reset_out3/1 -> psi_d/1, Sum33/2(In2)
  From8/1 -> Product9/2(In2)
  Mux_in_pipe3/1 -> mux2/4
  Mux_in_pipe4/1 -> mux2/5
  Product1_outbuff/1 -> Sum1_stage2/2(In2)
  Product7_outbuff/1 -> Sum1_stage3/2(In2)
  reset_out2/1 -> psi_q/1, Sum31/2(In2)
  reset_integrators1/1 -> reset_out2/2, reset_out3/2, reset_in3/2, reset_in2/2
  Switch11/1 -> Goto5/1, Product/1(In1)
  reset_out1/1 -> delayMatch2/1, theta_el/1
  From2/1 -> delayMatch3/1, reset_out1/2
  Product4_outbuff/1 -> Sum/2(In2)
  delayMatch8/1 -> Sum1/1(In1)
  delayMatch5/1 -> Switch11/2
  Data Type Conversion3/1(Out1) -> t2/1
  Data Type Conversion15/1(Out1) -> Mux_in_pipe1/1
  Data Type Conversion6/1(Out1) -> Data Type Conversion6_out1_in_pipe/1
  Product8/1(Out1) -> Product8_outbuff/1
  Data Type Conversion7/1(Out1) -> Data Type Conversion7_out1_in_pipe/1
  Data Type Conversion9/1(Out1) -> Data Type Conversion9_out1_in_pipe/1
  Sum2/1(Out1) -> Sum2_outbuff/1
  Product5/1(Out1) -> Product5_outbuff/1
  Product2/1(Out1) -> Product2_outbuff/1
  Product1/1(Out1) -> Product1_outbuff/1
  Data Type Conversion21/1(Out1) -> t3/1
  Data Type Conversion17/1(Out1) -> Mux_in_pipe3/1
  Data Type Conversion2/1(Out1) -> t4/1
  Data Type Conversion20/1(Out1) -> Mux_in_pipe4/1
  Sum/1(Out1) -> Sum_outbuff/1
  Data Type Conversion12/1(Out1) -> Product12/1(In1)
  Abs/1(Out1) -> Abs_outbuff/1
  Product12/1(Out1) -> Product12_outbuff/1
  Data Type Conversion13/1(Out1) -> Sum5/2(In2)
  Sum5/1(Out1) -> Sum5_outbuff/1
  Product4/1(Out1) -> Product4_outbuff/1
  Sign1/1(Out1) -> Sign1_outbuff/1
  Data Type Conversion14/1(Out1) -> Product11/1(In1)
  Data Type Conversion4/1(Out1) -> Switch11/3
  Data Type Conversion5/1(Out1) -> Sum1/2(In2)
  Sum1/1(Out1) -> Sum1_outbuff/1
  Product11/1(Out1) -> Product11_outbuff/1
  Sum3/1(Out1) -> Sum3_outbuff/1
  Compare To Constant1_relop/1(Out1) -> Compare To Constant1_relop_outbuff/1
  Sum11/1(Out1) -> Sum1_outbuff1/1
  Sum21/1(Out1) -> Sum2_outbuff1/1
  Compare To Constant_relop/1(Out1) -> Compare To Constant_relop_outbuff/1
  Sum4/1(Out1) -> Sum_outbuff1/1
  Data Type Conversion10/1(Out1) -> Data Type Conversion10_out1_in_pipe/1
  Product/1(Out1) -> Gain1/2(In2)
  Product10/1(Out1) -> Product10_outbuff/1
  Product3/1(Out1) -> Product_outbuff/1
  Sum31/1(Out1) -> Sum3_outbuff1/1
  Sum1_stage2/1(Out1) -> Sum1_stage2_outbuff/1
  Sum1_stage3/1(Out1) -> Sum1_stage3_outbuff/1
  Product7/1(Out1) -> Product7_outbuff/1
  Data Type Conversion8/1(Out1) -> Data Type Conversion8_out1_in_pipe/1
  Product6/1(Out1) -> Product6_outbuff/1
  Data Type Conversion11/1(Out1) -> Mux_in_pipe0/1
  Data Type Conversion16/1(Out1) -> Mux_in_pipe2/1
  Product9/1(Out1) -> Product9_outbuff/1
  Sum32/1(Out1) -> Sum3_outbuff2/1
  Product31/1(Out1) -> Product3_outbuff/1
  Sum33/1(Out1) -> Sum3_outbuff3/1
  Sum_stage2/1(Out1) -> Sum_stage2_outbuff/1
  Sum_stage3/1(Out1) -> Sum_stage3_outbuff/1
  Data Type Conversion19/1(Out1) -> t5/1
  Data Type Conversion18/1(Out1) -> Data Type Conversion18_out_pipe/1
  Data Type Conversion1/1(Out1) -> Data Type Conversion1_out_pipe/1
  Gain/1(Out1) -> Gain_outbuff/1
  Gain1/1(Out1) -> Sum4/2(In2)
  Gain2/1(Out1) -> Gain_outbuff1/1
  Factor/1(Out1) -> Factor_outbuff/1
  Gain3/1(Out1) -> Gain_outbuff2/1
  mechanical_system_out1/1 -> delayMatch4/1
  Data Type Conversion10_out1/1 -> Goto4/1, Product10/2(In2)
  psi_q/1 -> Product6/1(In1), pmsm_out4/1, Product3/2(In2)
  pmsm_out3_out_pipe/1 -> Product31/1(In1)
  pmsm_out4_out_pipe/1 -> Product2/2(In2)
  Product3_outbuff/1 -> Sum32/1(In1)
  Mux_in_pipe0/1 -> mux2/1
  Mux_in_pipe1/1 -> mux2/2
  From5/1 -> mux1/2
  psi_d/1 -> Sum2/1(In1), pmsm_out3/1, Product1/2(In2)
  Data Type Conversion6_out1/1 -> Product8/2(In2), Product7/2(In2)
  From9/1 -> Product/2(In2)
  delayMatch2/1 -> Sum4/1(In1)
  Compare To Constant_relop_outbuff/1 -> Switch/2
  Sum_outbuff1/1 -> Compare To Constant_relop/1(In1), Sum11/1(In1), Switch/3
  Compare To Constant1_relop_outbuff/1 -> Switch1/2
  Switch/1 -> Sum21/2(In2), Compare To Constant1_relop/1(In1), Switch1/3
  delayMatch3/1 -> reset_in1/2
  Abs_outbuff/1 -> delayMatch6/1
  Sign1_outbuff/1 -> delayMatch7/1
  reset_out/1 -> delayMatch9/1, integrator1_out1/1
  From1/1 -> delayMatch10/1, reset_out/2

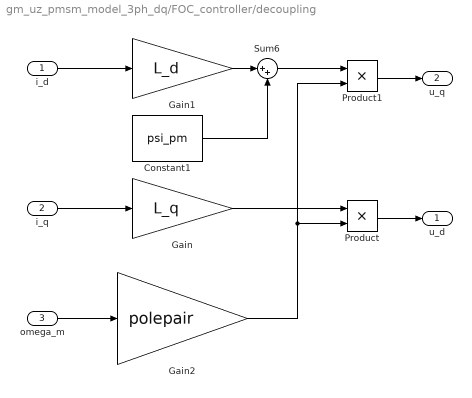
== system gm_uz_pmsm_model_3ph_dq/FOC_controller/decoupling ==
  i_d : Inport
  i_q : Inport  Port=2
  omega_m : Inport  Port=3
  Constant1 : Constant  Value=psi_pm  SampleTime=-1
  Gain : Gain  Gain=L_q
  Gain1 : Gain  Gain=L_d
  Gain2 : Gain  Gain=polepair
  Product : Product
  Product1 : Product
  Sum6 : Sum  Inputs=|++
  u_d : Outport
  u_q : Outport  Port=2
  wires:
  omega_m/1 -> Gain2/1
  Sum6/1 -> Product1/1
  Constant1/1 -> Sum6/2
  i_q/1 -> Gain/1
  Gain1/1 -> Sum6/1
  Product/1 -> u_d/1
  i_d/1 -> Gain1/1
  Product1/1 -> u_q/1
  Gain2/1 -> Product/2, Product1/2
  Gain/1 -> Product/1

== system gm_uz_pmsm_model_3ph_dq/uz_pmsm_model_3ph_dq/Abs ==
  In1 : Inport
  Abs : Abs  SampleTime=1e-08  OutDataTypeStr=double
  Out1 : Outport
  wires:
  In1/1 -> Abs/1
  Abs/1 -> Out1/1

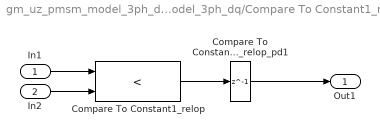
== system gm_uz_pmsm_model_3ph_dq/uz_pmsm_model_3ph_dq/Compare To Constant1_relop ==
  In1 : Inport
  In2 : Inport  Port=2
  Compare To Constant1_relop : RelationalOperator  Operator=<  OutDataTypeStr=boolean  SampleTime=1e-08  RndMeth=Nearest  InputSameDT=on
  Compare To Constant1_relop_pd1 : Delay  DelayLength=1
  Out1 : Outport
  wires:
  In1/1 -> Compare To Constant1_relop/1
  In2/1 -> Compare To Constant1_relop/2
  Compare To Constant1_relop/1 -> Compare To Constant1_relop_pd1/1
  Compare To Constant1_relop_pd1/1 -> Out1/1

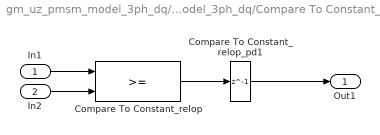
== system gm_uz_pmsm_model_3ph_dq/uz_pmsm_model_3ph_dq/Compare To Constant_relop ==
  In1 : Inport
  In2 : Inport  Port=2
  Compare To Constant_relop : RelationalOperator  OutDataTypeStr=boolean  SampleTime=1e-08  RndMeth=Nearest  InputSameDT=on
  Compare To Constant_relop_pd1 : Delay  DelayLength=1
  Out1 : Outport
  wires:
  In1/1 -> Compare To Constant_relop/1
  In2/1 -> Compare To Constant_relop/2
  Compare To Constant_relop/1 -> Compare To Constant_relop_pd1/1
  Compare To Constant_relop_pd1/1 -> Out1/1

== system gm_uz_pmsm_model_3ph_dq/uz_pmsm_model_3ph_dq/Data Type Conversion1 ==
  In1 : Inport
  Data Type Conversion1 : DataTypeConversion  OutDataTypeStr=double  RndMeth=Nearest  SampleTime=1e-08
  Data Type Conversion1_pd1 : Delay  DelayLength=3
  Out1 : Outport
  wires:
  In1/1 -> Data Type Conversion1/1
  Data Type Conversion1/1 -> Data Type Conversion1_pd1/1
  Data Type Conversion1_pd1/1 -> Out1/1

== system gm_uz_pmsm_model_3ph_dq/uz_pmsm_model_3ph_dq/Data Type Conversion10 ==
  In1 : Inport
  Data Type Conversion10 : DataTypeConversion  OutDataTypeStr=double  RndMeth=Nearest  SampleTime=1e-08
  Data Type Conversion10_pd1 : Delay  DelayLength=3
  Out1 : Outport
  wires:
  In1/1 -> Data Type Conversion10/1
  Data Type Conversion10/1 -> Data Type Conversion10_pd1/1
  Data Type Conversion10_pd1/1 -> Out1/1

== system gm_uz_pmsm_model_3ph_dq/uz_pmsm_model_3ph_dq/Data Type Conversion11 ==
  In1 : Inport
  Data Type Conversion11 : DataTypeConversion  OutDataTypeStr=single  RndMeth=Nearest  SampleTime=1e-08
  Data Type Conversion11_pd1 : Delay  DelayLength=3
  Out1 : Outport
  wires:
  In1/1 -> Data Type Conversion11/1
  Data Type Conversion11/1 -> Data Type Conversion11_pd1/1
  Data Type Conversion11_pd1/1 -> Out1/1

== system gm_uz_pmsm_model_3ph_dq/uz_pmsm_model_3ph_dq/Data Type Conversion12 ==
  In1 : Inport
  Data Type Conversion12 : DataTypeConversion  OutDataTypeStr=double  RndMeth=Nearest  SampleTime=1e-08
  Data Type Conversion12_pd1 : Delay  DelayLength=3
  Out1 : Outport
  wires:
  In1/1 -> Data Type Conversion12/1
  Data Type Conversion12/1 -> Data Type Conversion12_pd1/1
  Data Type Conversion12_pd1/1 -> Out1/1

== system gm_uz_pmsm_model_3ph_dq/uz_pmsm_model_3ph_dq/Data Type Conversion13 ==
  In1 : Inport
  Data Type Conversion13 : DataTypeConversion  OutDataTypeStr=double  RndMeth=Nearest  SampleTime=1e-08
  Data Type Conversion13_pd1 : Delay  DelayLength=3
  Out1 : Outport
  wires:
  In1/1 -> Data Type Conversion13/1
  Data Type Conversion13/1 -> Data Type Conversion13_pd1/1
  Data Type Conversion13_pd1/1 -> Out1/1

== system gm_uz_pmsm_model_3ph_dq/uz_pmsm_model_3ph_dq/Data Type Conversion14 ==
  In1 : Inport
  Data Type Conversion14 : DataTypeConversion  OutDataTypeStr=double  RndMeth=Nearest  SampleTime=1e-08
  Data Type Conversion14_pd1 : Delay  DelayLength=3
  Out1 : Outport
  wires:
  In1/1 -> Data Type Conversion14/1
  Data Type Conversion14/1 -> Data Type Conversion14_pd1/1
  Data Type Conversion14_pd1/1 -> Out1/1

== system gm_uz_pmsm_model_3ph_dq/uz_pmsm_model_3ph_dq/Data Type Conversion15 ==
  In1 : Inport
  Data Type Conversion15 : DataTypeConversion  OutDataTypeStr=single  RndMeth=Nearest  SampleTime=1e-08
  Data Type Conversion15_pd1 : Delay  DelayLength=3
  Out1 : Outport
  wires:
  In1/1 -> Data Type Conversion15/1
  Data Type Conversion15/1 -> Data Type Conversion15_pd1/1
  Data Type Conversion15_pd1/1 -> Out1/1

== system gm_uz_pmsm_model_3ph_dq/uz_pmsm_model_3ph_dq/Data Type Conversion16 ==
  In1 : Inport
  Data Type Conversion16 : DataTypeConversion  OutDataTypeStr=single  RndMeth=Nearest  SampleTime=1e-08
  Data Type Conversion16_pd1 : Delay  DelayLength=3
  Out1 : Outport
  wires:
  In1/1 -> Data Type Conversion16/1
  Data Type Conversion16/1 -> Data Type Conversion16_pd1/1
  Data Type Conversion16_pd1/1 -> Out1/1

== system gm_uz_pmsm_model_3ph_dq/uz_pmsm_model_3ph_dq/Data Type Conversion17 ==
  In1 : Inport
  Data Type Conversion17 : DataTypeConversion  OutDataTypeStr=single  RndMeth=Nearest  SampleTime=1e-08
  Data Type Conversion17_pd1 : Delay  DelayLength=3
  Out1 : Outport
  wires:
  In1/1 -> Data Type Conversion17/1
  Data Type Conversion17/1 -> Data Type Conversion17_pd1/1
  Data Type Conversion17_pd1/1 -> Out1/1

== system gm_uz_pmsm_model_3ph_dq/uz_pmsm_model_3ph_dq/Data Type Conversion18 ==
  In1 : Inport
  Data Type Conversion18 : DataTypeConversion  OutDataTypeStr=double  RndMeth=Nearest  SampleTime=1e-08
  Data Type Conversion18_pd1 : Delay  DelayLength=3
  Out1 : Outport
  wires:
  In1/1 -> Data Type Conversion18/1
  Data Type Conversion18/1 -> Data Type Conversion18_pd1/1
  Data Type Conversion18_pd1/1 -> Out1/1

== system gm_uz_pmsm_model_3ph_dq/uz_pmsm_model_3ph_dq/Data Type Conversion19 ==
  In1 : Inport
  Data Type Conversion19 : DataTypeConversion  OutDataTypeStr=single  RndMeth=Nearest  SampleTime=1e-08
  Data Type Conversion19_pd1 : Delay  DelayLength=3
  Out1 : Outport
  wires:
  In1/1 -> Data Type Conversion19/1
  Data Type Conversion19/1 -> Data Type Conversion19_pd1/1
  Data Type Conversion19_pd1/1 -> Out1/1

== system gm_uz_pmsm_model_3ph_dq/uz_pmsm_model_3ph_dq/Data Type Conversion2 ==
  In1 : Inport
  Data Type Conversion2 : DataTypeConversion  OutDataTypeStr=fixdt(1, 18, 14)  RndMeth=Nearest  SampleTime=1e-08
  Data Type Conversion2_pd1 : Delay  DelayLength=3
  Out1 : Outport
  wires:
  In1/1 -> Data Type Conversion2/1
  Data Type Conversion2/1 -> Data Type Conversion2_pd1/1
  Data Type Conversion2_pd1/1 -> Out1/1

== system gm_uz_pmsm_model_3ph_dq/uz_pmsm_model_3ph_dq/Data Type Conversion20 ==
  In1 : Inport
  Data Type Conversion20 : DataTypeConversion  OutDataTypeStr=single  RndMeth=Nearest  SampleTime=1e-08
  Data Type Conversion20_pd1 : Delay  DelayLength=3
  Out1 : Outport
  wires:
  In1/1 -> Data Type Conversion20/1
  Data Type Conversion20/1 -> Data Type Conversion20_pd1/1
  Data Type Conversion20_pd1/1 -> Out1/1

== system gm_uz_pmsm_model_3ph_dq/uz_pmsm_model_3ph_dq/Data Type Conversion21 ==
  In1 : Inport
  Data Type Conversion21 : DataTypeConversion  OutDataTypeStr=fixdt(1, 24, 11)  RndMeth=Nearest  SampleTime=1e-08
  Data Type Conversion21_pd1 : Delay  DelayLength=3
  Out1 : Outport
  wires:
  In1/1 -> Data Type Conversion21/1
  Data Type Conversion21/1 -> Data Type Conversion21_pd1/1
  Data Type Conversion21_pd1/1 -> Out1/1

== system gm_uz_pmsm_model_3ph_dq/uz_pmsm_model_3ph_dq/Data Type Conversion3 ==
  In1 : Inport
  Data Type Conversion3 : DataTypeConversion  OutDataTypeStr=fixdt(1, 27, 18)  RndMeth=Nearest  SampleTime=1e-08
  Data Type Conversion3_pd1 : Delay  DelayLength=3
  Out1 : Outport
  wires:
  In1/1 -> Data Type Conversion3/1
  Data Type Conversion3/1 -> Data Type Conversion3_pd1/1
  Data Type Conversion3_pd1/1 -> Out1/1

== system gm_uz_pmsm_model_3ph_dq/uz_pmsm_model_3ph_dq/Data Type Conversion4 ==
  In1 : Inport
  Data Type Conversion4 : DataTypeConversion  OutDataTypeStr=double  RndMeth=Nearest  SampleTime=1e-08
  Data Type Conversion4_pd1 : Delay  DelayLength=3
  Out1 : Outport
  wires:
  In1/1 -> Data Type Conversion4/1
  Data Type Conversion4/1 -> Data Type Conversion4_pd1/1
  Data Type Conversion4_pd1/1 -> Out1/1
